simulink model "DCPM_motor_and_Pendulum"  (R2023b)
settings: Solver=VariableStepAuto  StartTime=0.0  StopTime=30  RelTol=1e-3
values from neighbouring files (symbols this model uses):
  alfa = 1e-5    (= 1e-05)    [consistent.m]
  alfa_10 = 1.034391e-5    (= 1.034391e-05)    [consistent.m]
  alfa_11 = 9.64721e-6    (= 9.64721e-06)    [consistent.m]
  alfa_12 = 1.46e-5    (= 1.46e-05)    [consistent.m]
  beta = 1.295e-5    (= 1.295e-05)    [consistent.m]
  g0 = 9.81    [consistent.m]    (also in dyn_model.m)
  Ip = (mp*Lp^2)/12    (= 3.3282e-05)    [consistent.m]    (also in dyn_model.m = 8.3205e-06)
  Ip_tot = (mp*(Lp/2)^2)+Ip    (= 0.000133128)    [consistent.m]
  Ir = 9.6e-5    (= 9.6e-05)    [consistent.m]    (also in dyn_model.m = 1.42994791667e-05)
  Ir_tot = Ir+J+J_hub    (= 0.0001006)    [consistent.m]
  J = 4e-6    (= 4e-06)    [consistent.m]    (also in dyn_model.m)
  J_hub = 0.6e-6    (= 6e-07)    [consistent.m]
  K = place(A,B,P)    [consistent.m]
  La = 1.16e-3    (= 0.00116)    [consistent.m]    (also in dyn_model.m)
  Lp = 0.129    [consistent.m]    (also in dyn_model.m = 0.0645)
  Lr = 0.085    [consistent.m]    (also in dyn_model.m)
  mp = 0.024    [consistent.m]    (also in dyn_model.m)
  mr = 0.095    [consistent.m]    (also in dyn_model.m)
  phi_dot_init = 0    [consistent.m]
  phi_init_10 = 90    [consistent.m]
  phi_init_11 = 45    [consistent.m]
  phi_init_12 = 8.7891    [consistent.m]
  Ra = 8.4    [consistent.m]    (also in dyn_model.m)
  theta_dot_init = 0    [consistent.m]
  theta_init = 0    [consistent.m]
undefined symbols (not defined in the file or in its folder): rot_pend
libraries: simulink_extras x5
settings Model: PacingRate=1000  Creator=Mark  LastModifiedBy=Mark

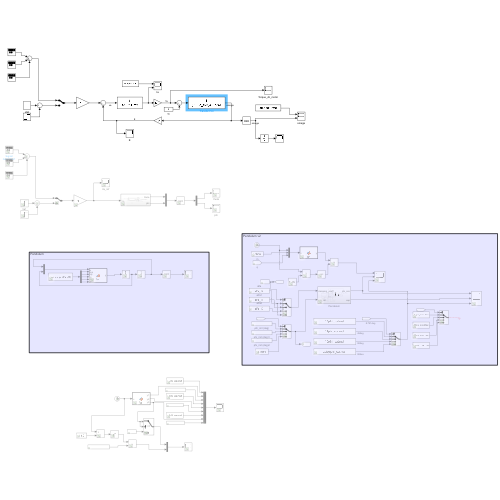
[thumbnail: Simulink's stored preview of the top-level diagram]
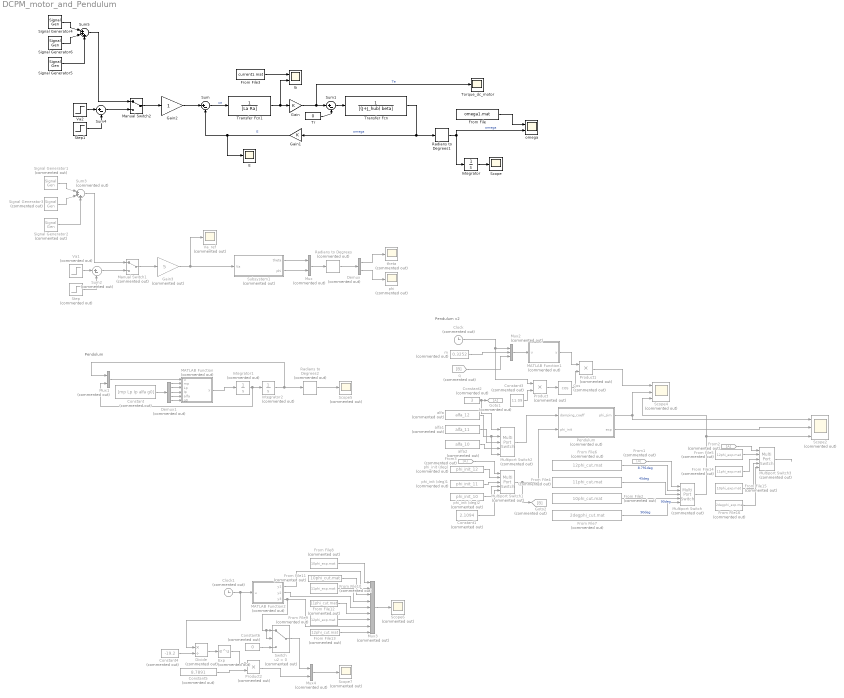
== system DCPM_motor_and_Pendulum ==
  note: Pendulum v2
  note: Pendolum
  Clock : Clock  Commented=on
  Clock1 : Clock  Commented=on
  Constant : Constant  Commented=on  Value=[mp Lp Ip alfa g0]
  Constant1 : Constant  Commented=on  Value=2.1094
  Constant2 : Constant  Commented=on  Value=3
  Constant3 : Constant  Commented=on  Value=11.09
  Constant4 : Constant  Commented=on  Value=-19.2
  Constant5 : Constant  Commented=on  Value=8.7891
  Constant6 : Constant  Commented=on  Value=0
  Cos : Trigonometry  Commented=on  Operator=cos
  Demux : Demux  Commented=on  Outputs=2
  Demux1 : Demux  Commented=on  Outputs=5
  Divide : Product  Commented=on  Inputs=*/
  E : Scope
  Exp : Math  Commented=on
  From File : FromFile  FileName=omega1.mat  SampleTime=0
  From File10 : FromFile  Commented=on  FileName=11phi_exp.mat  SampleTime=0
  From File11 : FromFile  Commented=on  FileName=10phi_cut.mat  SampleTime=0
  From File12 : FromFile  Commented=on  FileName=11phi_cut.mat  SampleTime=0
  From File13 : FromFile  Commented=on  FileName=12phi_cut.mat  SampleTime=0
  From File14 : FromFile  Commented=on  FileName=11phi_exp.mat  SampleTime=0
  From File15 : FromFile  Commented=on  FileName=10phi_exp.mat  SampleTime=0
  From File16 : FromFile  Commented=on  FileName=2degphi_exp.mat  SampleTime=0
  From File2 : FromFile  Commented=on  FileName=10phi_cut.mat  SampleTime=0
  From File3 : FromFile  FileName=current1.mat  SampleTime=0
  From File4 : FromFile  Commented=on  FileName=11phi_cut.mat  SampleTime=0
  From File5 : FromFile  Commented=on  FileName=12phi_exp.mat  SampleTime=0
  From File6 : FromFile  Commented=on  FileName=12phi_cut.mat  SampleTime=0
  From File7 : FromFile  Commented=on  FileName=2degphi_cut.mat  SampleTime=0
  From File8 : FromFile  Commented=on  FileName=10phi_exp.mat  SampleTime=0
  From File9 : FromFile  Commented=on  FileName=12phi_exp.mat  SampleTime=0
  From1 : From  Commented=on
  From2 : From  Commented=on
  From3 : From  Commented=on
  Gain : Gain  Gain=K
  Gain1 : Gain  Gain=K
  Gain2 : Gain
  Gain3 : Gain  Commented=on  Gain=5
  Goto1 : Goto  Commented=on
  Goto2 : Goto  Commented=on  GotoTag=B
  Ia : Scope  NumInputPorts=2
  Integrator : Integrator
  Integrator1 : Integrator  Commented=on
  Integrator2 : Integrator  Commented=on  InitialCondition=0.1534
  MATLAB Function : MATLAB Function  Commented=on  TreatAsAtomicUnit=on
  MATLAB Function1 : MATLAB Function  Commented=on  TreatAsAtomicUnit=on
  MATLAB Function2 : MATLAB Function  Commented=on  TreatAsAtomicUnit=on
  Manual Switch1 : ManualSwitch  Commented=on
  Manual Switch2 : ManualSwitch
  Multiport Switch{,1..3} (4 alike) : MultiPortSwitch  Commented=on  Inputs=4  SaturateOnIntegerOverflow=off  InputSameDT=off
  Mux : Mux  Commented=on  Inputs=2
  Mux1 : Mux  Commented=on  Inputs=2
  Mux2 : Mux  Commented=on  Inputs=3
  Mux3 : Mux  Commented=on  Inputs=9
  Mux4 : Mux  Commented=on  Inputs=2
  Pendulum : Subsystem  Commented=on
  Product : Product  Commented=on
  Product1 : Product  Commented=on
  Product2 : Product  Commented=on
  Radians to Degrees : simulink_extras/Transformations/Radians to Degrees  Commented=on
  Radians to Degrees1 : simulink_extras/Transformations/Radians to Degrees
  Radians to Degrees2 : simulink_extras/Transformations/Radians to Degrees  Commented=on
  Scope : Scope
  Scope2 : Scope  Commented=on  NumInputPorts=3
  Scope4 : Scope  Commented=on  NumInputPorts=3
  Scope5 : Scope  Commented=on
  Scope6 : Scope  Commented=on
  Scope7 : Scope  Commented=on
  Signal Generator1 : SignalGenerator  Commented=on  WaveForm=square  Frequency=0.25
  Signal Generator2 : SignalGenerator  Commented=on  WaveForm=square  Amplitude=0  Frequency=7
  Signal Generator3 : SignalGenerator  Commented=on  WaveForm=square  Amplitude=0  Frequency=5
  Signal Generator4 : SignalGenerator  WaveForm=square  Frequency=0.25
  Signal Generator5 : SignalGenerator  WaveForm=square  Amplitude=0  Frequency=7
  Signal Generator6 : SignalGenerator  WaveForm=square  Amplitude=0  Frequency=5
  Step : Step  Commented=on  Time=1.05  SampleTime=0
  Step1 : Step  Time=1.05  SampleTime=0
  Subsystem1 : Subsystem  Commented=on
  Sum : Sum  Inputs=|+-
  Sum1 : Sum  Inputs=|+-
  Sum2 : Sum  Commented=on  Inputs=|+-
  Sum3 : Sum  Commented=on  Inputs=|+++
  Sum4 : Sum  Inputs=|+-
  Sum5 : Sum  Inputs=|+++
  Switch : Switch  Commented=on  Criteria=u2 > Threshold  SaturateOnIntegerOverflow=off  InputSameDT=off
  Torque_dc_motor : Scope
  Tr : Constant  Value=0
  Transfer Fcn : TransferFcn  Denominator=[(J+J_hub) beta]
  Transfer Fcn1 : TransferFcn  Denominator=[La Ra]
  Va1 : Step  Commented=on  SampleTime=0
  Va2 : Step  SampleTime=0
  Va_ref : Scope  Commented=on
  alfa : Constant  Commented=on  Value=alfa_12
  alfa1 : Constant  Commented=on  Value=alfa_11
  alfa2 : Constant  Commented=on  Value=alfa_10
  m : Constant  Commented=on  Value=0.3252
  omega : Scope  NumInputPorts=2
  phi : Scope  Commented=on
  phi_init (deg) : Constant  Commented=on  Value=phi_init_12
  phi_init (deg)1 : Constant  Commented=on  Value=phi_init_11
  phi_init (deg)2 : Constant  Commented=on  Value=phi_init_10
  q : From  Commented=on  GotoTag=B
  theta : Scope  Commented=on
  wires:
  Tr/1 -> Sum1/2
  Sum/1 -> Transfer Fcn1/1  "ua"
  Gain1/1 -> E/1, Sum/2  "E"
  Transfer Fcn1/1 -> Ia/2, Gain/1
  Gain/1 -> Torque_dc_motor/1, Sum1/1  "Te"
  Sum1/1 -> Transfer Fcn/1
  Manual Switch1/1 -> Gain3/1
  Sum2/1 -> Manual Switch1/2
  Sum3/1 -> Manual Switch1/1
  Subsystem1/1(theta) -> Mux/1
  Subsystem1/2(phi) -> Mux/2
  Radians to Degrees/1 -> Demux/1
  Mux/1 -> Radians to Degrees/1
  Demux/1 -> theta/1
  Demux/2 -> phi/1
  Va1/1 -> Sum2/1
  Step/1 -> Sum2/2
  Gain2/1 -> Sum/1
  Integrator/1 -> Scope/1
  Transfer Fcn/1 -> Radians to Degrees1/1, Gain1/1  "omega"
  Radians to Degrees1/1 -> omega/2, Integrator/1  "omega"
  MATLAB Function/1(y) -> Integrator1/1
  Integrator1/1 -> Integrator2/1, Mux1/2
  Integrator2/1 -> Mux1/1, Radians to Degrees2/1
  Signal Generator1/1 -> Sum3/1
  Signal Generator3/1 -> Sum3/2
  Signal Generator2/1 -> Sum3/3
  Radians to Degrees2/1 -> Scope5/1
  Mux1/1 -> MATLAB Function/1(u)
  Demux1/1 -> MATLAB Function/2(mp)
  Demux1/2 -> MATLAB Function/3(Lp)
  Demux1/3 -> MATLAB Function/4(Ip)
  Demux1/4 -> MATLAB Function/5(alfa)
  Constant/1 -> Demux1/1
  Demux1/5 -> MATLAB Function/6(g0)
  From File/1 -> omega/1
  From File3/1 -> Ia/1
  From File2/1 -> Multiport Switch/4  "90deg"
  From File4/1 -> Multiport Switch/3  "45deg"
  From File6/1 -> Multiport Switch/2  "8.791deg"
  Multiport Switch/1 -> Scope4/3, Scope2/3
  From File5/1 -> Multiport Switch3/2
  phi_init (deg)/1 -> Multiport Switch1/2
  Pendulum/1(phi_sim) -> Scope2/1, Scope4/2
  alfa/1 -> Multiport Switch2/5, Multiport Switch2/2
  phi_init (deg)1/1 -> Multiport Switch1/3
  phi_init (deg)2/1 -> Multiport Switch1/4
  From1/1 -> Multiport Switch/1
  From3/1 -> Multiport Switch1/1
  Multiport Switch1/1 -> Goto2/1, Pendulum/2(phi_init)
  alfa2/1 -> Multiport Switch2/4
  alfa1/1 -> Multiport Switch2/3
  Constant2/1 -> Multiport Switch2/1, Goto1/1
  Multiport Switch2/1 -> Pendulum/1(damping_coeff)
  Constant1/1 -> Multiport Switch1/5
  From File7/1 -> Multiport Switch/5  "90deg"
  Clock/1 -> Product/1, Mux2/1
  Constant3/1 -> Product/2
  Product/1 -> Cos/1
  Cos/1 -> Product1/2
  MATLAB Function1/1(y) -> Product1/1
  Product1/1 -> Scope4/1
  q/1 -> Mux2/3
  Mux2/1 -> MATLAB Function1/1(u)
  m/1 -> Mux2/2
  Mux3/1 -> Scope6/1
  From File8/1 -> Mux3/1
  From File10/1 -> Mux3/4
  From File9/1 -> Mux3/7
  MATLAB Function2/1(y1) -> Mux3/2
  MATLAB Function2/2(y2) -> Mux3/5
  MATLAB Function2/3(y3) -> Switch/2, Switch/1, Mux3/8
  Clock1/1 -> Divide/1, MATLAB Function2/1(u)
  From File11/1 -> Mux3/3
  From File12/1 -> Mux3/6
  From File13/1 -> Mux3/9
  Constant4/1 -> Divide/2
  Divide/1 -> Exp/1
  Exp/1 -> Product2/1
  Constant5/1 -> Product2/2
  Mux4/1 -> Scope7/1
  Product2/1 -> Mux4/2
  Constant6/1 -> Switch/3
  Switch/1 -> Mux4/1
  From2/1 -> Multiport Switch3/1
  From File14/1 -> Multiport Switch3/3
  From File15/1 -> Multiport Switch3/4
  From File16/1 -> Multiport Switch3/5
  Multiport Switch3/1 -> ?
  Pendulum/2(exp) -> Scope2/2
  Gain3/1 -> Subsystem1/1(Va), Va_ref/1
  Sum4/1 -> Manual Switch2/2
  Signal Generator6/1 -> Sum5/2
  Signal Generator5/1 -> Sum5/3
  Step1/1 -> Sum4/2
  Signal Generator4/1 -> Sum5/1
  Manual Switch2/1 -> Gain2/1
  Sum5/1 -> Manual Switch2/1
  Va2/1 -> Sum4/1

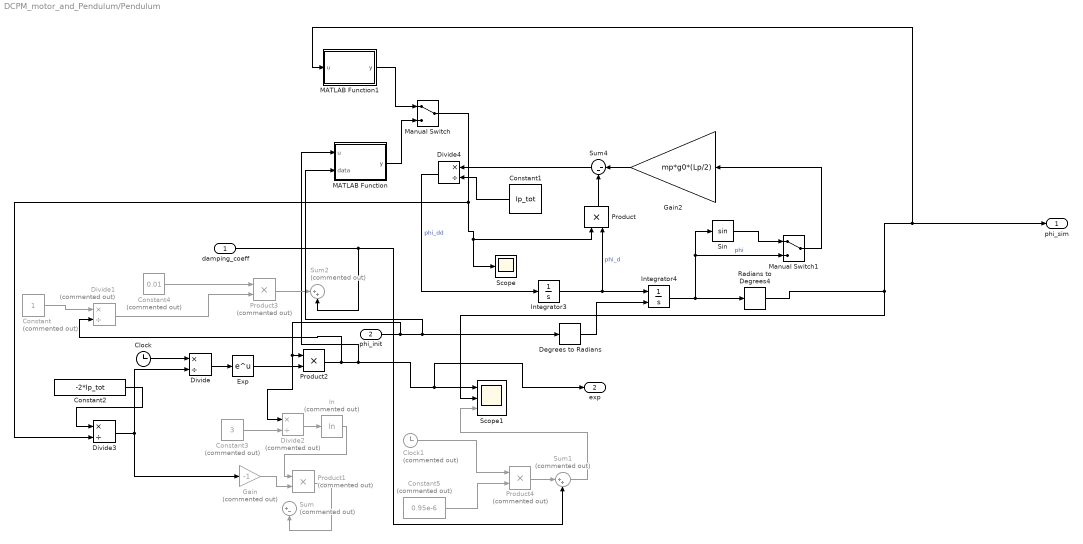
== system DCPM_motor_and_Pendulum/Pendulum ==
  damping_coeff : Inport
  phi_init : Inport  Port=2
  Clock : Clock
  Clock1 : Clock  Commented=on
  Constant : Constant  Commented=on
  Constant1 : Constant  Value=Ip_tot
  Constant2 : Constant  Value=-2*Ip_tot
  Constant3 : Constant  Commented=on  Value=3
  Constant4 : Constant  Commented=on  Value=0.01
  Constant5 : Constant  Commented=on  Value=0.95e-6
  Degrees to Radians : simulink_extras/Transformations/Degrees to Radians
  Divide : Product  Inputs=*/
  Divide1 : Product  Commented=on  Inputs=*/
  Divide2 : Product  Commented=on  Inputs=*/
  Divide3 : Product  Inputs=*/
  Divide4 : Product  Inputs=*/
  Exp : Math
  Gain : Gain  Commented=on  Gain=-1
  Gain2 : Gain  Gain=mp*g0*(Lp/2)
  Integrator3 : Integrator
  Integrator4 : Integrator  InitialConditionSource=external
  MATLAB Function : MATLAB Function  TreatAsAtomicUnit=on
  MATLAB Function1 : MATLAB Function  TreatAsAtomicUnit=on
  Manual Switch : ManualSwitch
  Manual Switch1 : ManualSwitch
  Product : Product
  Product1 : Product  Commented=on
  Product2 : Product
  Product3 : Product  Commented=on
  Product4 : Product  Commented=on
  Radians to Degrees4 : simulink_extras/Transformations/Radians to Degrees
  Scope : Scope
  Scope1 : Scope  NumInputPorts=3
  Sin : Trigonometry
  Sum : Sum  Commented=on  Inputs=|+-
  Sum1 : Sum  Commented=on  Inputs=|++
  Sum2 : Sum  Commented=on  Inputs=|++
  Sum4 : Sum  Inputs=|--
  ln : Math  Commented=on  Operator=log
  phi_sim : Outport
  exp : Outport  Port=2
  wires:
  Integrator4/1 -> Manual Switch1/2, Sin/1, Radians to Degrees4/1  "phi"
  Sum4/1 -> Divide4/1
  Gain2/1 -> Sum4/1
  Product/1 -> Sum4/2
  Integrator3/1 -> Integrator4/1, Product/2  "phi_d"
  Constant1/1 -> Divide4/2
  Degrees to Radians/1 -> Integrator4/2
  Radians to Degrees4/1 -> Scope1/2, MATLAB Function1/1(u), phi_sim/1
  damping_coeff/1 -> Sum1/2, Sum2/2
  Clock/1 -> Divide/1
  Divide/1 -> Exp/1
  Exp/1 -> Product2/2
  Product2/1 -> Divide1/2, MATLAB Function/1(u), exp/1, Scope1/1
  Constant4/1 -> Product3/1
  Product3/1 -> Sum2/1
  Constant/1 -> Divide1/1
  Divide1/1 -> Product3/2
  phi_init/1 -> Divide2/1, Product2/1, MATLAB Function/2(data), Degrees to Radians/1
  Constant3/1 -> Divide2/2
  Divide2/1 -> ln/1
  ln/1 -> Product1/1
  Gain/1 -> Product1/2
  Product1/1 -> Sum/2
  Clock1/1 -> Product4/1
  Constant5/1 -> Product4/2
  Product4/1 -> Sum1/1
  Sum1/1 -> Scope1/3
  Constant2/1 -> Divide3/1
  Divide3/1 -> Divide/2, Gain/1
  Divide4/1 -> Integrator3/1  "phi_dd"
  Manual Switch/1 -> Scope/1, Product/1, Divide3/2
  MATLAB Function/1(y) -> Manual Switch/2
  MATLAB Function1/1(y) -> Manual Switch/1
  Manual Switch1/1 -> Gain2/1
  Sin/1 -> Manual Switch1/1

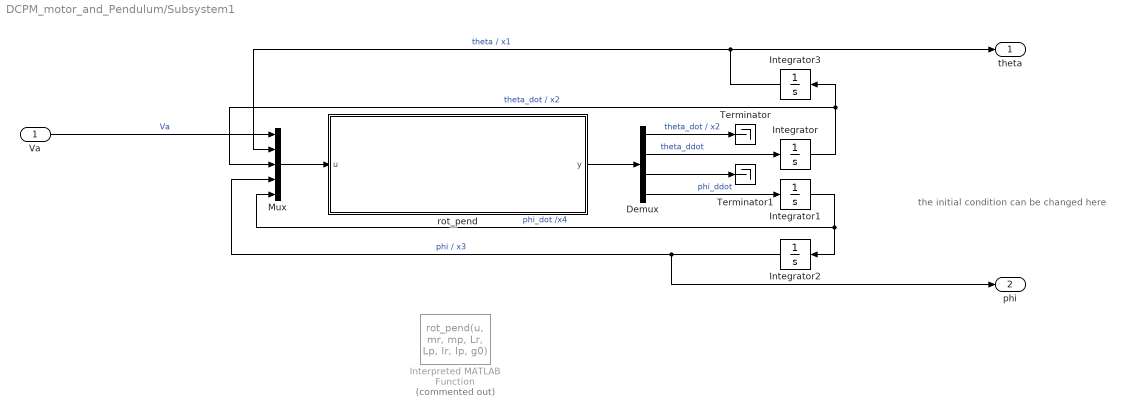
== system DCPM_motor_and_Pendulum/Subsystem1 ==
  note: the initial condition can be changed here
  Va : Inport
  Demux : Demux
  Integrator : Integrator  InitialCondition=theta_dot_init
  Integrator1 : Integrator  InitialCondition=phi_dot_init
  Integrator2 : Integrator  InitialCondition=pi/4
  Integrator3 : Integrator  InitialCondition=theta_init
  Interpreted MATLAB Function : MATLABFcn  Commented=on  MATLABFcn=rot_pend(u, mr, mp, Lr, Lp, Ir, Ip, g0)  OutputDimensions=4  OutputSignalType=real
  Mux : Mux  Inputs=5
  Terminator : Terminator
  Terminator1 : Terminator
  rot_pend : Subsystem
  theta : Outport
  phi : Outport  Port=2
  wires:
  Integrator2/1 -> phi/1, Mux/4  "phi / x3"
  Integrator/1 -> Mux/3, Integrator3/1  "theta_dot / x2"
  Mux/1 -> rot_pend/1(u)
  rot_pend/1(y) -> Demux/1
  Integrator1/1 -> Mux/5, Integrator2/1  "phi_dot /x4"
  Integrator3/1 -> theta/1, Mux/2  "theta / x1"
  Demux/4 -> Integrator1/1  "phi_ddot"
  Demux/2 -> Integrator/1  "theta_ddot"
  Demux/1 -> Terminator/1  "theta_dot / x2"
  Demux/3 -> Terminator1/1
  Va/1 -> Mux/1  "Va"

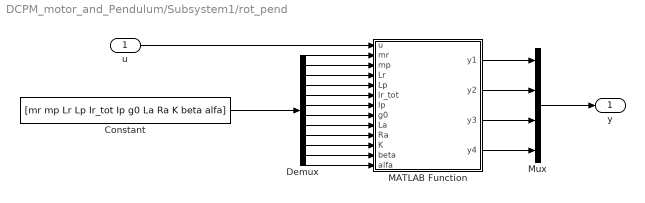
== system DCPM_motor_and_Pendulum/Subsystem1/rot_pend ==
  u : Inport
  Constant : Constant  Value=[mr mp Lr Lp Ir_tot Ip g0 La Ra K beta alfa]  VectorParams1D=off
  Demux : Demux  Outputs=12
  MATLAB Function : MATLAB Function  TreatAsAtomicUnit=on
  Mux : Mux
  y : Outport
  wires:
  Demux/3 -> MATLAB Function/4(Lr)
  Demux/5 -> MATLAB Function/6(Ir_tot)
  Demux/4 -> MATLAB Function/5(Lp)
  Demux/7 -> MATLAB Function/8(g0)
  Demux/2 -> MATLAB Function/3(mp)
  Demux/6 -> MATLAB Function/7(Ip)
  Demux/1 -> MATLAB Function/2(mr)
  u/1 -> MATLAB Function/1(u)
  Constant/1 -> Demux/1
  MATLAB Function/1(y1) -> Mux/1
  MATLAB Function/2(y2) -> Mux/2
  MATLAB Function/3(y3) -> Mux/3
  MATLAB Function/4(y4) -> Mux/4
  Mux/1 -> y/1
  Demux/8 -> MATLAB Function/9(La)
  Demux/9 -> MATLAB Function/10(Ra)
  Demux/10 -> MATLAB Function/11(K)
  Demux/11 -> MATLAB Function/12(beta)
  Demux/12 -> MATLAB Function/13(alfa)

== matlab function DCPM_motor_and_Pendulum/Subsystem1/rot_pend/MATLAB Function ==
  data: u input; y1 output; mr input; mp input; Lr input; Lp input; Ir_tot input; Ip input; g0 input; La input; Ra input; y2 output; y3 output; y4 output; K input; beta input; alfa input
function [y1,y2,y3,y4] = rot_pend(u, mr, mp, Lr, Lp, Ir_tot, Ip, g0,La, Ra, K, beta, alfa)
%UNTITLED Summary of this function goes here
%   Detailed explanation goes here
% u(1) = Va
x1 = u(2) ; % theta
x2 = u(3) ; % theta_dot
x3 = u(4) ; % phi
x4 = u(5) ; % phi_dot

H = [(mp*(Lr^2+((Lp/2)^2*(sin(x3))^2)))+Ir_tot            -mp*Lr*Lp*cos(x3)/2;
                     -mp*Lr*Lp*cos(x3)/2                              (mp*(Lp/2)^2)+Ip] ;

Q = [mp*(Lp/2)^2*sin(x3)*cos(x3)*x4+beta                      (mp*(Lp/2)^2*sin(x3)*cos(x3)*x2)-(mp*Lr*(Lp/2)*sin(x3)*x4);
     -mp*(Lp/2)^2*sin(x3)*cos(x3)*x2                                                   alfa                                   ] ;

g = [           0     ;
     mp*g0*(Lp/2)*sin(x3)] ;
%(K*u(1)/Ra)-(K^2*x2/Ra)
tau = [(K*u(1)/Ra)-(K^2*x2/Ra);
       0 ] ;
 % Fv = [beta 0;
 %         0   alfa] ;
q_ddot = H\[tau - Q*[x2 x4]' - g ] ;



y1 = x2 ;
y2 = q_ddot(1) ;
y3 = x4 ;
y4 = q_ddot(2) ;


%Ir+mr*(Lr/2)^2)

== matlab function DCPM_motor_and_Pendulum/MATLAB Function ==
  data: u input; y output; mp input; Lp input; Ip input; alfa input; g0 input
function y = fcn(u, mp, Lp, Ip, alfa, g0)
I = (mp*(Lp/2)^2)+Ip ;
y = -( (mp*g0*(Lp/2)*sin(u(1))) + (alfa*u(2)) ) / I;

== matlab function DCPM_motor_and_Pendulum/MATLAB Function2 ==
  data: u input; y1 output; y2 output; y3 output
function [y1,y2,y3] = fcn(u)

y1 = - (4.6875*u) + 90 ;
y2 = - (3.1394*u) + 45;
y3 = - (1.2129*u) + 8.7891 ;

== matlab function DCPM_motor_and_Pendulum/MATLAB Function1 ==
  data: u input; y output
function y = fcn(u)

y = - (u(2)*u(1)) + u(3);

== matlab function DCPM_motor_and_Pendulum/Pendulum/MATLAB Function ==
  data: u input; y output; data input
function y = fcn(u, data)
if data>=10
    if u>=45
        y = 1e-5 ;
    elseif u<45 && u>=(0.2*data)
        y = 1.25e-5 ;
    elseif u<(0.2*data) && u>=(0.1*data)
        y = 2e-5 ;
    else
        y = 3e-5 ;
    end
else
    if u>=4
        y = 1.46e-5 ;
    elseif u<4 && u>=2
        y = 2e-5 ;
    else
        y = 3e-5 ;
    end
end

== matlab function DCPM_motor_and_Pendulum/Pendulum/MATLAB Function1 ==
  data: u input; y output
function y = fcn(u)
% if u>=10
%     y = 1.46e-6 ;
% elseif u<10 && u>=2
%     y = 1.46e-5 ;
% else
%     y = 1.8e-5 ;
% 
% end

y = 1e-5 ;
